simulink model "burst_hwc"  (R2015a)
settings: Solver=ode45  StartTime=0.0  StopTime=NUM_SIM_CYCLES  RelTol=1e-3
values from neighbouring files (symbols this model uses):
  STEP_SIZE = 328    [run_sg_burst_hwc.m]
libraries: xbsIndex_r4 x12, dspbuff3 x3
settings Model: CovSFcnEnable=off  Creator=bwiec  LastModifiedBy=bwiec
settings DebuggingCC: SolverPrmCheckMsg=warning

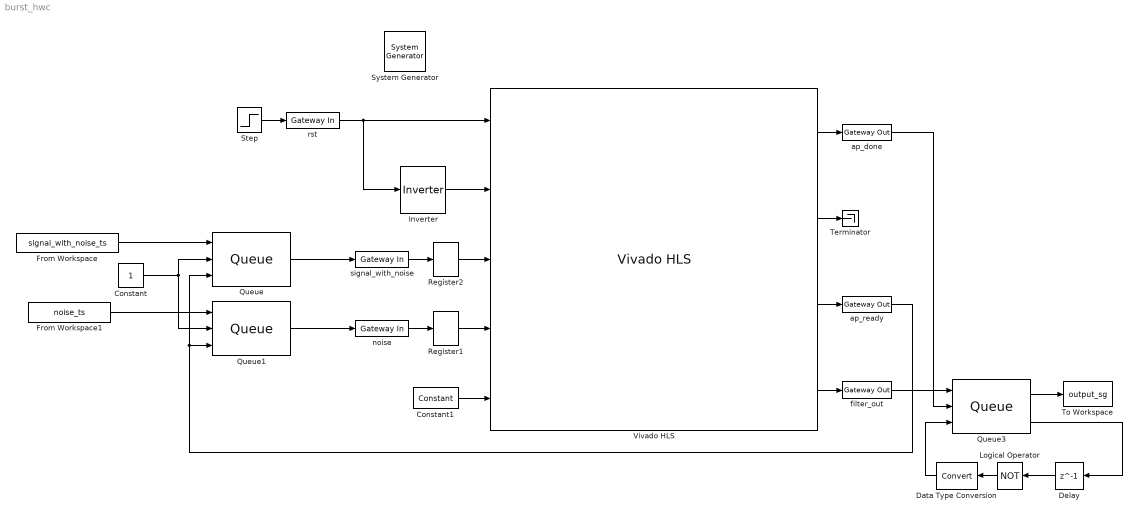
== system burst_hwc ==
  " System Generator" : xbsIndex_r4/ System Generator  Tag=genX  xilinxfamily=kintex7  part=xc7k325t  speed=-2  package=ffg900  synthesis_tool=Vivado  clock_wrapper=Clock Enables  directory=./netlist  proj_type=Vivado  Synth_file=Vivado Synthesis Defaults  Impl_file=Vivado Implementation Defaults  testbench=off  simulink_period=1  sysclk_period=20  dcm_input_clock_period=10  incr_netlist=off  trim_vbits=Everywhere in SubSystem  dbl_ovrd=According to Block Masks  core_generation=According to Block Masks  run_coregen=off  deprecated_control=off  eval_field=0  block_type=sysgen
  Constant : Constant
  Constant1 : xbsIndex_r4/Constant  const=STEP_SIZE  gui_display_data_type=Fixed-point  arith_type=Signed (2's comp)  n_bits=16  bin_pt=0  preci_type=Single  exp_width=8  frac_width=24  explicit_period=on  period=1  equ=P=C  opselect=C  inp2=PCIN>>17  opr=+  inp1=P  carry=CIN  dbl_ovrd=off  block_type=constant
  Data Type Conversion : DataTypeConversion
  Delay : Delay  DelayLength=1  InitialCondition=0
  From Workspace : FromWorkspace  VariableName=signal_with_noise_ts  SampleTime=1
  From Workspace1 : FromWorkspace  VariableName=noise_ts  SampleTime=1
  Inverter : xbsIndex_r4/Inverter  en=off  latency=1  dbl_ovrd=off  block_type=inv
  Logical Operator : Logic  Operator=NOT  AllPortsSameDT=off  OutDataTypeStr=boolean
  Queue : dspbuff3/Queue  depth=65536  trigger=Non-zero sample  overflow=Dynamic reallocation  pes=Warning  eso=off  fso=off  nso=off  clr=off  clrOutport=off  adf=on
  Queue1 : dspbuff3/Queue  depth=65536  trigger=Non-zero sample  overflow=Dynamic reallocation  pes=Warning  eso=off  fso=off  nso=off  clr=off  clrOutport=off  adf=on
  Queue3 : dspbuff3/Queue  depth=65536  trigger=Non-zero sample  overflow=Dynamic reallocation  pes=Warning  eso=on  fso=off  nso=off  clr=off  clrOutport=off  adf=on
  Register1 : xbsIndex_r4/Register  init=0  rst=off  en=off  dbl_ovrd=off  block_type=register
  Register2 : xbsIndex_r4/Register  init=0  rst=off  en=off  dbl_ovrd=off  block_type=register
  Step : Step  Time=10  Before=1  After=0  SampleTime=0
  Terminator : Terminator
  To Workspace : ToWorkspace  VariableName=output_sg  SaveFormat=Timeseries  SampleTime=-1
  Vivado HLS : xbsIndex_r4/Vivado HLS  anytable='../vhls/proj/hls_adaptive_filter_v1_0/max_throughput'  fast_sim=on  display_datatype=on  rate_propagation_method=Simulink system period  model_file_path=''  latency=1  block_type=hls
      settings: infoedit=This block allows including C,C++ and SystemC source files in System Generator for DSP designs.
  ap_done : xbsIndex_r4/Gateway Out  inherit_from_input=off  hdl_port=on  rows=1  columns=1  UseAsDAC=off  DACChannel='1'  interface=None  automatic_assignment=on  address_offset=hex2dec('00')  intf_name=''  intf_description=''  timing_constraint=None  locs_specified=off  LOCs={}  io_standard={}  block_type=gatewayout
  ap_ready : xbsIndex_r4/Gateway Out  inherit_from_input=off  hdl_port=on  rows=1  columns=1  UseAsDAC=off  DACChannel='1'  interface=None  automatic_assignment=on  address_offset=hex2dec('00')  intf_name=''  intf_description=''  timing_constraint=None  locs_specified=off  LOCs={}  io_standard={}  block_type=gatewayout
  filter_out : xbsIndex_r4/Gateway Out  inherit_from_input=off  hdl_port=on  rows=1  columns=1  UseAsDAC=off  DACChannel='1'  interface=None  automatic_assignment=on  address_offset=hex2dec('00')  intf_name=''  intf_description=''  timing_constraint=None  locs_specified=off  LOCs={}  io_standard={}  block_type=gatewayout
  noise : xbsIndex_r4/Gateway In  gui_display_data_type=Fixed-point  arith_type="Signed  (2's comp)"  n_bits=16  bin_pt=0  preci_type=Single  exp_width=8  frac_width=24  rows=1  columns=1  quantization="Round  (unbiased: +/- Inf)"  overflow=Saturate  period=1  UseAsADC=off  ADCChannel='1'  interface=None  automatic_assignment=on  address_offset=hex2dec('00')  intf_name=''  intf_description=''  timing_constraint=None  locs_specified=off  LOCs={}  io_standard={}  inherit_from_input=off  hdl_port=on  dbl_ovrd=off  block_type=gatewayin
  rst : xbsIndex_r4/Gateway In  gui_display_data_type=Boolean  arith_type=Boolean  n_bits=16  bin_pt=14  preci_type=Single  exp_width=8  frac_width=24  rows=1  columns=1  quantization="Round  (unbiased: +/- Inf)"  overflow=Saturate  period=1  UseAsADC=off  ADCChannel='1'  interface=None  automatic_assignment=on  address_offset=hex2dec('00')  intf_name=''  intf_description=''  timing_constraint=None  locs_specified=off  LOCs={}  io_standard={}  inherit_from_input=off  hdl_port=on  dbl_ovrd=off  block_type=gatewayin
  signal_with_noise : xbsIndex_r4/Gateway In  gui_display_data_type=Fixed-point  arith_type="Signed  (2's comp)"  n_bits=16  bin_pt=0  preci_type=Single  exp_width=8  frac_width=24  rows=1  columns=1  quantization="Round  (unbiased: +/- Inf)"  overflow=Saturate  period=1  UseAsADC=off  ADCChannel='1'  interface=None  automatic_assignment=on  address_offset=hex2dec('00')  intf_name=''  intf_description=''  timing_constraint=None  locs_specified=off  LOCs={}  io_standard={}  inherit_from_input=off  hdl_port=on  dbl_ovrd=off  block_type=gatewayin
  wires:
  Step/1 -> rst/1
  rst/1 -> Inverter/1, Vivado HLS/1
  Inverter/1 -> Vivado HLS/2
  signal_with_noise/1 -> Register2/1
  noise/1 -> Register1/1
  Vivado HLS/3 -> ap_ready/1
  Vivado HLS/4 -> filter_out/1
  Vivado HLS/1 -> ap_done/1
  Vivado HLS/2 -> Terminator/1
  Constant1/1 -> Vivado HLS/5
  Register1/1 -> Vivado HLS/4
  Register2/1 -> Vivado HLS/3
  From Workspace/1 -> Queue/1
  Queue/1 -> signal_with_noise/1
  Constant/1 -> Queue1/2, Queue/2
  ap_ready/1 -> Queue1/3, Queue/3
  From Workspace1/1 -> Queue1/1
  Queue1/1 -> noise/1
  filter_out/1 -> Queue3/1
  Queue3/1 -> To Workspace/1
  ap_done/1 -> Queue3/2
  Queue3/2 -> Delay/1
  Logical Operator/1 -> Data Type Conversion/1
  Data Type Conversion/1 -> Queue3/3
  Delay/1 -> Logical Operator/1
